simulink library "MM5"  (R2024a)
settings: Solver=VariableStepAuto  StartTime=0.0  StopTime=10.0  RelTol=1e-3
undefined symbols (not defined in the file or in its folder): raptor_xcp_function, StateCAN
libraries: Utilities x16, Raptor_lib x6, simulink x1
settings Model: Creator=serga  LastModifiedBy=hyuga
settings ConfigComp: CovBoundaryAbsTol=1.0e-5

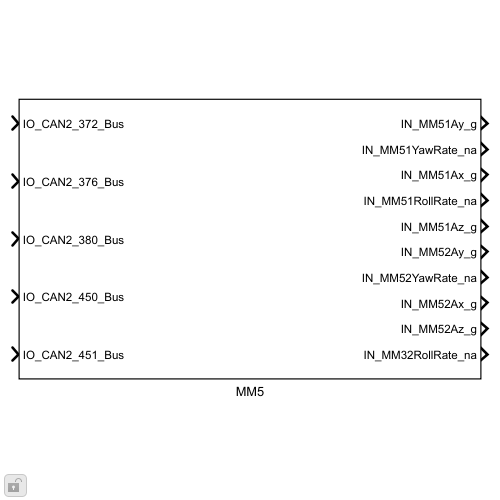
[thumbnail: Simulink's stored preview of the top-level diagram]
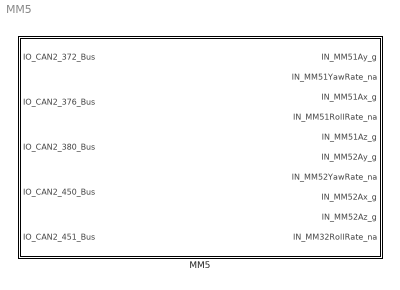
== system MM5 ==
  MM5 : Subsystem

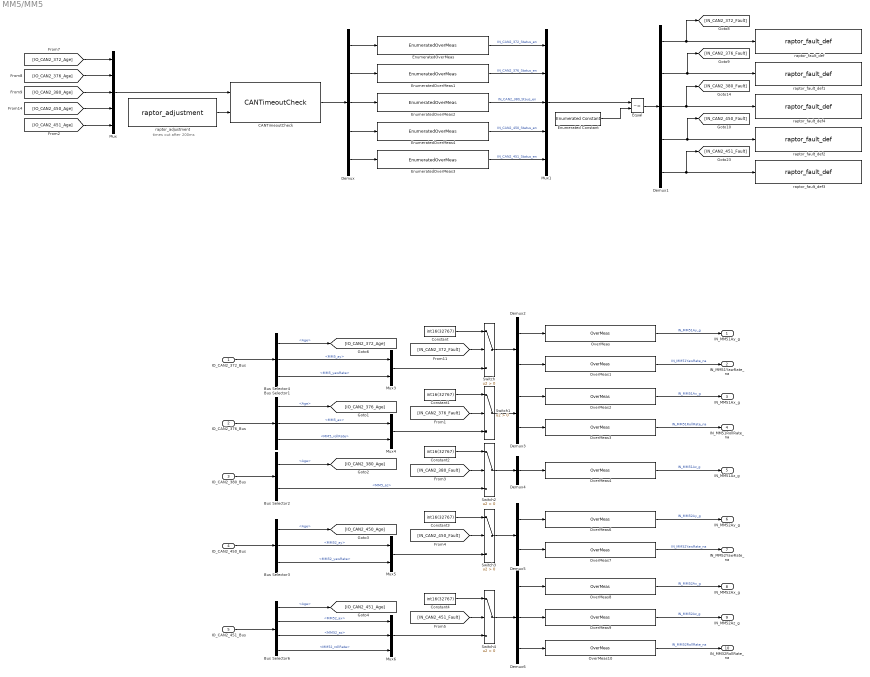
== system MM5/MM5 ==
  note: times out after 200ms
  IO_CAN2_372_Bus : Inport
  IO_CAN2_376_Bus : Inport  Port=2
  IO_CAN2_380_Bus : Inport  Port=3
  IO_CAN2_450_Bus : Inport  Port=4
  IO_CAN2_451_Bus : Inport  Port=5
  Bus Selector1 : BusSelector  OutputSignals=Age,MM5_ax,MM5_rollRate
  Bus Selector2 : BusSelector  OutputSignals=Age,MM5_az
  Bus Selector3 : BusSelector  OutputSignals=Age,MM52_ay,MM52_yawRate
  Bus Selector4 : BusSelector  OutputSignals=Age,MM5_ay,MM5_yawRate
  Bus Selector6 : BusSelector  OutputSignals=Age,MM52_ax,MM52_az,MM52_rollRate
  CANTimeoutCheck : Utilities/CANTimeoutCheck
  Constant{,1..4} (5 alike) : Constant  Value=int16(32767)
  Demux : Demux  Outputs=5
  Demux1 : Demux  Outputs=5
  Demux2 : Demux  Outputs=2
  Demux3 : Demux  Outputs=2
  Demux4 : Demux  Outputs=1
  Demux5 : Demux  Outputs=2
  Demux6 : Demux  Outputs=3
  Enumerated Constant : simulink/Sources/Enumerated Constant  OutDataTypeStr=Enum: StateCAN  Value=StateCAN.Normal  SampleTime=inf
  EnumeratedOverMeas : Utilities/EnumeratedOverMeas  sigName='IN_CAN2_372_Status_en'  enumName='StateCAN'
  EnumeratedOverMeas1 : Utilities/EnumeratedOverMeas  sigName='IN_CAN2_376_Status_en'  enumName='StateCAN'
  EnumeratedOverMeas2 : Utilities/EnumeratedOverMeas  sigName='IN_CAN2_380_Staus_en'  enumName='StateCAN'
  EnumeratedOverMeas3 : Utilities/EnumeratedOverMeas  sigName='IN_CAN2_451_Status_en'  enumName='StateCAN'
  EnumeratedOverMeas4 : Utilities/EnumeratedOverMeas  sigName='IN_CAN2_450_Status_en'  enumName='StateCAN'
  Equal : RelationalOperator  Operator=~=  OutDataTypeStr=boolean  RndMeth=Simplest  InputSameDT=off
  Mux : Mux  Inputs=5
  Mux1 : Mux  Inputs=5
  Mux3 : Mux  Inputs=2
  Mux4 : Mux  Inputs=2
  Mux5 : Mux  Inputs=2
  Mux6 : Mux  Inputs=3
  OverMeas : Utilities/OverMeas  sigName='IN_MM51Ay_g'  minimum=-inf  maximum=inf
  OverMeas1 : Utilities/OverMeas  sigName='IN_MM51YawRate_na'  minimum=-inf  maximum=inf
  OverMeas10 : Utilities/OverMeas  sigName='IN_MM52RollRate_na'  minimum=-inf  maximum=inf
  OverMeas2 : Utilities/OverMeas  sigName='IN_MM51Ax_g'  minimum=-inf  maximum=inf
  OverMeas3 : Utilities/OverMeas  sigName='IN_MM51RollRate_na'  minimum=-inf  maximum=inf
  OverMeas4 : Utilities/OverMeas  sigName='IN_MM51Az_g'  minimum=-inf  maximum=inf
  OverMeas6 : Utilities/OverMeas  sigName='IN_MM52Ay_g'  minimum=-inf  maximum=inf
  OverMeas7 : Utilities/OverMeas  sigName='IN_MM52YawRate_na'  minimum=-inf  maximum=inf
  OverMeas8 : Utilities/OverMeas  sigName='IN_MM52Ax_g'  minimum=-inf  maximum=inf
  OverMeas9 : Utilities/OverMeas  sigName='IN_MM52Az_g'  minimum=-inf  maximum=inf
  Switch{,1..4} (5 alike) : Switch  Criteria=u2 > Threshold  SaturateOnIntegerOverflow=off  InputSameDT=off
  raptor_adjustment : Raptor_lib/Data Storage/raptor_adjustment  paramName='IN_MM5TOThresh_na'  nameSource=Parameter  initValue=20  dataType=int32  storage=Calibration  calDispType=Number  calEnum={'False', 'True'}  calGain=1.0  calOffset=0.0  calMax=inf  calMin=-inf  calFormat='-1'  calUnit=''  calHelp=''  calAccess=1  calFunction=raptor_xcp_function(gcb)  calDispHeaders=off  calColHeaders={'Col1' 'Col2' 'Col3'}  calRowHeaders={'Row1' 'Row2' 'Row3'}
      settings: SourceProductName=Raptor
  raptor_fault_def : Raptor_lib/Faults/raptor_fault_def  faultName='IN_CAN2_372_Fault'  persist=on  sticky=off  emisRelated=off  permanent=off  singleTrip=off  clearMethod=Standard  xLimit=25  yLimit=50  calEnable=on  addDisable=off  calAccess=1  calFunction='System | FaultManager'
      settings: SourceProductName=Raptor
  raptor_fault_def1 : Raptor_lib/Faults/raptor_fault_def  faultName='IN_CAN2_376_Fault'  persist=on  sticky=off  emisRelated=off  permanent=off  singleTrip=off  clearMethod=Standard  xLimit=25  yLimit=50  calEnable=on  addDisable=off  calAccess=1  calFunction='System | FaultManager'
      settings: SourceProductName=Raptor
  raptor_fault_def2 : Raptor_lib/Faults/raptor_fault_def  faultName='IN_CAN2_450_Fault'  persist=on  sticky=off  emisRelated=off  permanent=off  singleTrip=off  clearMethod=Standard  xLimit=25  yLimit=50  calEnable=on  addDisable=off  calAccess=1  calFunction='System | FaultManager'
      settings: SourceProductName=Raptor
  raptor_fault_def3 : Raptor_lib/Faults/raptor_fault_def  faultName='IN_CAN2_451_Fault'  persist=on  sticky=off  emisRelated=off  permanent=off  singleTrip=off  clearMethod=Standard  xLimit=25  yLimit=50  calEnable=on  addDisable=off  calAccess=1  calFunction='System | FaultManager'
      settings: SourceProductName=Raptor
  raptor_fault_def4 : Raptor_lib/Faults/raptor_fault_def  faultName='IN_CAN2_380_Fault'  persist=on  sticky=off  emisRelated=off  permanent=off  singleTrip=off  clearMethod=Standard  xLimit=25  yLimit=50  calEnable=on  addDisable=off  calAccess=1  calFunction='System | FaultManager'
      settings: SourceProductName=Raptor
  IN_MM51Ay_g : Outport
  IN_MM51YawRate_na : Outport  Port=2
  IN_MM51Ax_g : Outport  Port=3
  IN_MM51RollRate_na : Outport  Port=4
  IN_MM51Az_g : Outport  Port=5
  IN_MM52Ay_g : Outport  Port=6
  IN_MM52YawRate_na : Outport  Port=7
  IN_MM52Ax_g : Outport  Port=8
  IN_MM52Az_g : Outport  Port=9
  IN_MM32RollRate_na : Outport  Port=10
  wires:
  Equal/1 -> Demux1/1
  Demux1/3 -> [IN_CAN2_380_Fault], raptor_fault_def4/1
  [IO_CAN2_380_Age] -> Mux/3
  EnumeratedOverMeas3/1 -> Mux1/5  "IN_CAN2_451_Status_en"
  raptor_adjustment/1 -> CANTimeoutCheck/2
  Enumerated Constant/1 -> Equal/2
  Demux1/4 -> [IN_CAN2_450_Fault], raptor_fault_def2/1
  Demux/1 -> EnumeratedOverMeas/1
  Mux/1 -> CANTimeoutCheck/1
  EnumeratedOverMeas4/1 -> Mux1/4  "IN_CAN2_450_Status_en"
  Demux/4 -> EnumeratedOverMeas4/1
  [IO_CAN2_372_Age] -> Mux/1
  Demux/5 -> EnumeratedOverMeas3/1
  Demux1/1 -> [IN_CAN2_372_Fault], raptor_fault_def/1
  Demux1/5 -> [IN_CAN2_451_Fault], raptor_fault_def3/1
  Demux1/2 -> [IN_CAN2_376_Fault], raptor_fault_def1/1
  Demux/3 -> EnumeratedOverMeas2/1
  Mux1/1 -> Equal/1
  Demux/2 -> EnumeratedOverMeas1/1
  EnumeratedOverMeas/1 -> Mux1/1  "IN_CAN2_372_Status_en"
  CANTimeoutCheck/1 -> Demux/1
  [IO_CAN2_450_Age] -> Mux/4
  [IO_CAN2_376_Age] -> Mux/2
  EnumeratedOverMeas1/1 -> Mux1/2  "IN_CAN2_376_Status_en"
  EnumeratedOverMeas2/1 -> Mux1/3  "IN_CAN2_380_Staus_en"
  Switch/1 -> Demux2/1
  Demux2/2 -> OverMeas1/1
  Demux2/1 -> OverMeas/1
  Mux3/1 -> Switch/3
  [IN_CAN2_372_Fault] -> Switch/2
  OverMeas1/1 -> IN_MM51YawRate_na/1  "IN_MM51YawRate_na"
  Bus Selector4/1 -> [IO_CAN2_372_Age]  "<Age>"
  Constant/1 -> Switch/1
  OverMeas/1 -> IN_MM51Ay_g/1  "IN_MM51Ay_g"
  IO_CAN2_372_Bus/1 -> Bus Selector4/1
  Bus Selector4/2 -> Mux3/1  "<MM5_ay>"
  Bus Selector4/3 -> Mux3/2  "<MM5_yawRate>"
  IO_CAN2_376_Bus/1 -> Bus Selector1/1
  OverMeas2/1 -> IN_MM51Ax_g/1  "IN_MM51Ax_g"
  Constant1/1 -> Switch1/1
  Bus Selector1/1 -> [IO_CAN2_376_Age]  "<Age>"
  OverMeas3/1 -> IN_MM51RollRate_na/1  "IN_MM51RollRate_na"
  [IN_CAN2_376_Fault] -> Switch1/2
  Mux4/1 -> Switch1/3
  Demux3/1 -> OverMeas2/1
  Demux3/2 -> OverMeas3/1
  Switch1/1 -> Demux3/1
  Bus Selector1/2 -> Mux4/1  "<MM5_ax>"
  Bus Selector1/3 -> Mux4/2  "<MM5_rollRate>"
  Switch2/1 -> Demux4/1
  Demux4/1 -> OverMeas4/1
  [IN_CAN2_380_Fault] -> Switch2/2
  Bus Selector2/1 -> [IO_CAN2_380_Age]  "<Age>"
  Constant2/1 -> Switch2/1
  OverMeas4/1 -> IN_MM51Az_g/1  "IN_MM51Az_g"
  IO_CAN2_380_Bus/1 -> Bus Selector2/1
  Bus Selector2/2 -> Switch2/3  "<MM5_az>"
  Switch3/1 -> Demux5/1
  Demux5/1 -> OverMeas6/1
  [IN_CAN2_450_Fault] -> Switch3/2
  Demux5/2 -> OverMeas7/1
  IO_CAN2_450_Bus/1 -> Bus Selector3/1
  Mux5/1 -> Switch3/3
  OverMeas6/1 -> IN_MM52Ay_g/1  "IN_MM52Ay_g"
  OverMeas7/1 -> IN_MM52YawRate_na/1  "IN_MM52YawRate_na"
  Constant3/1 -> Switch3/1
  Bus Selector3/1 -> [IO_CAN2_450_Age]  "<Age>"
  Bus Selector3/2 -> Mux5/1  "<MM52_ay>"
  Bus Selector3/3 -> Mux5/2  "<MM52_yawRate>"
  OverMeas8/1 -> IN_MM52Ax_g/1  "IN_MM52Ax_g"
  Constant4/1 -> Switch4/1
  Bus Selector6/1 -> [IO_CAN2_451_Age]  "<Age>"
  OverMeas9/1 -> IN_MM52Az_g/1  "IN_MM52Az_g"
  [IN_CAN2_451_Fault] -> Switch4/2
  Mux6/1 -> Switch4/3
  Demux6/1 -> OverMeas8/1
  Demux6/2 -> OverMeas9/1
  Switch4/1 -> Demux6/1
  IO_CAN2_451_Bus/1 -> Bus Selector6/1
  Bus Selector6/2 -> Mux6/1  "<MM52_ax>"
  Bus Selector6/3 -> Mux6/2  "<MM52_az>"
  Bus Selector6/4 -> Mux6/3  "<MM52_rollRate>"
  Demux6/3 -> OverMeas10/1
  OverMeas10/1 -> IN_MM32RollRate_na/1  "IN_MM52RollRate_na"
  [IO_CAN2_451_Age] -> Mux/5
